simulink model "TrackerSingleObject"  (Simulink 8.4)
settings: Solver=FixedStepDiscrete  StartTime=0.0  StopTime=inf  RelTol=1e-3
libraries: instrumentlib x1
settings Model: Creator=Ssubrama  LastModifiedBy=kpetersen
settings OptimizationCC: InitFltsAndDblsToZero=on
settings GRTTargetCC: TargetFcnLib=ansi_tfl_tmw_new.mat

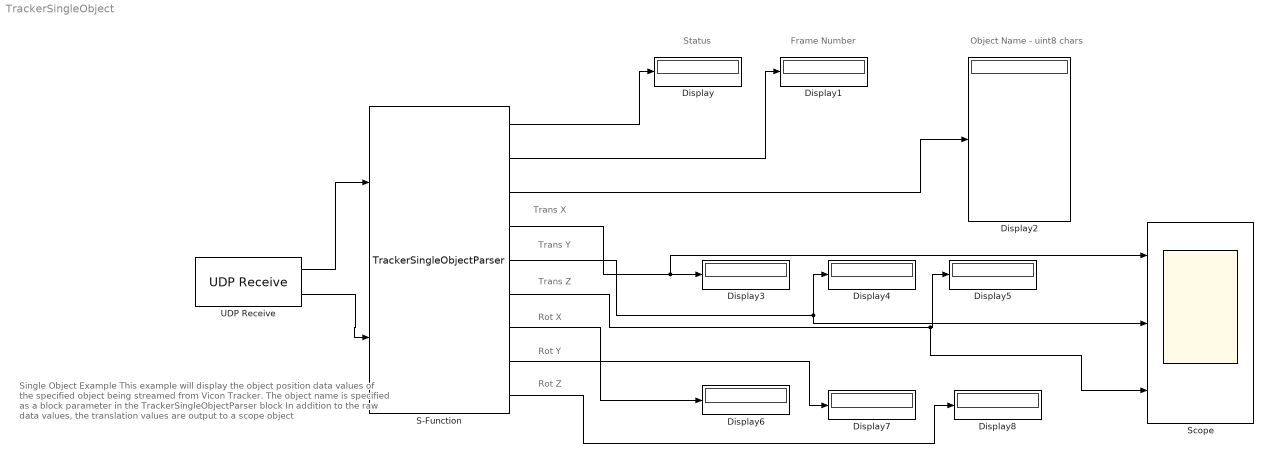
== system TrackerSingleObject ==
  note: Rot Z
  note: Rot Y
  note: Rot X
  note: Trans Z
  note: Trans Y
  note: Trans X
  note: Single Object Example
      |
      | This example will display the object position data
      | values of the specified object being streamed from
      | Vicon Tracker.
      |
      | The object name is specified as a block parameter
      | in the TrackerSingleObjectParser block
      |
      | In addition to the raw data values, the
      | translation values are output to a scope object
  note: Object Name - uint8 chars
  note: Frame Number
  note: Status
  Display{,1..8} (9 alike) : Display
  S-Function : S-Function  FunctionName=TrackerSingleObjectParser  Parameters='Object1'  SFunctionModules=TrackerSingleObjectParser  EnableBusSupport=off
      settings: AttributesFormatString=Data Parser
  Scope : Scope  NumInputPorts=3
      settings: YMin=0.4~-4~0.8  YMax=0.8~4~1  MaxDataPoints=200  SampleInput=on  ScrollMode=on
  UDP Receive : instrumentlib/UDP Receive  Priority=3  Host=localhost  Port=51001  LocalPort=51001  DataSize=256  EnableBlockingMode=off  Timeout=inf  SampleTime=0.01  DataType=uint8  ByteOrder=BigEndian
  wires:
  UDP Receive/1 -> S-Function/1
  S-Function/1 -> Display/1
  UDP Receive/2 -> S-Function/2
  S-Function/2 -> Display1/1
  S-Function/3 -> Display2/1
  S-Function/5 -> Display4/1, Scope/2
  S-Function/6 -> Scope/3, Display5/1
  S-Function/7 -> Display6/1
  S-Function/8 -> Display7/1
  S-Function/9 -> Display8/1
  S-Function/4 -> Scope/1, Display3/1
